simulink model "slave_exec"  (Simulink 3.00)
libraries: execlib x6

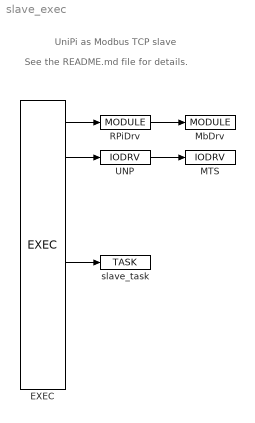
== system slave_exec ==
  note: UniPi as Modbus TCP slave
  note: See the README.md file for details.
  EXEC : execlib/EXEC  target=Generic target device  tick=0.005  ntick0=1  ntick1=50  ntick2=100  ntick3=1200  pri0=5  pri1=9  pri2=13  pri3=18
  MTS : execlib/IODRV  module=MbDrv  classname=MtsDrv  cfgname=slave_cfg.rio  factor=1  stack=10240  pri=3  timer=off
  MbDrv : execlib/MODULE
  RPiDrv : execlib/MODULE
  UNP : execlib/IODRV  module=RPiDrv  classname=UnpDrv  factor=1  stack=10240  pri=3  timer=off
  slave_task : execlib/TASK  factor=1  start=0  stop=1  stack=10240  MDLOPEN=on
  wires:
  EXEC/1 -> RPiDrv/1
  EXEC/2 -> UNP/1
  EXEC/5 -> slave_task/1
  RPiDrv/1 -> MbDrv/1
  UNP/1 -> MTS/1
